simulink model "PAM"  (R2020b)
settings: Solver=VariableStepAuto  StartTime=0.0  StopTime=10.0  RelTol=1e-3
settings Model: Creator=MRUNMAYEE J. MORE  LastModifiedBy=MRUNMAYEE J. MORE

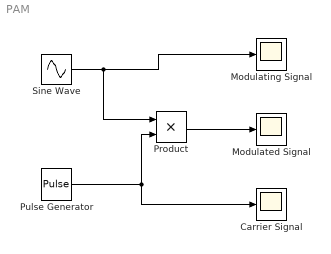
== system PAM ==
  Carrier Signal : Scope
  Modulated Signal : Scope
  Modulating Signal : Scope
  Product : Product
  Pulse Generator : DiscretePulseGenerator  PulseType=Time based  Period=0.2  PulseWidth=20
  Sine Wave : Sin  Amplitude=5  SampleTime=0.1
  wires:
  Sine Wave/1 -> Modulating Signal/1, Product/1
  Pulse Generator/1 -> Carrier Signal/1, Product/2
  Product/1 -> Modulated Signal/1
